simulink model "getAcceleration"  (R2019a)
settings: Solver=FixedStepAuto  StartTime=0.0  StopTime=inf  RelTol=1e-3  EnableMultiTasking=on
settings Model: SimulationMode=external  Creator=florian  LastModifiedBy=florian
settings SolverCC: PositivePriorityOrder=on
settings OptimizationCC: EnhancedBackFolding=on  PassReuseOutputArgsAs=Individual arguments  MaxStackSize=64  OptimizeBlockOrder=speed  DifferentSizesBufferReuse=on  OptimizationCustomize=off
settings DebuggingCC: ParameterTunabilityLossMsg=error
settings HardwareCC: ProdBitPerPointer=32  ProdBitPerSizeT=32  ProdBitPerPtrDiffT=32  ProdLargestAtomicInteger=Long  ProdLargestAtomicFloat=Double  ProdWordSize=32  ProdLongLongMode=on  ProdHWDeviceType=ARM Compatible->ARM Cortex
settings SFSimCC: MATLABDynamicMemAlloc=off
settings RTWCC: SystemTargetFile=ert.tlc  HardwareBoard=Raspberry Pi  TLCOptions="-aInlineSetEventsForThisBaseRateFcn=TLC_FALSE -aSuppressMultiTaskScheduler=TLC_FALSE  -aRateBasedStepFcn=0"  TemplateMakefile=ert_default_tmf  GenerateReport=on  Toolchain=GNU GCC Raspberry Pi  BuildConfiguration=Faster Runs  IncludeHyperlinkInReport=on  LaunchReport=on  GenerateTraceInfo=on  GenerateTraceReport=on  GenerateTraceReportSl=on  GenerateTraceReportSf=on  GenerateTraceReportEml=on
settings CodeAppCC: ForceParamTrailComments=on  IgnoreCustomStorageClasses=off  OperatorAnnotations=on  SimulinkDataObjDesc=on  SFDataObjDesc=on  InsertBlockDesc=on
settings ERTTargetCC: SupportContinuousTime=on  SupportVariableSizeSignals=on

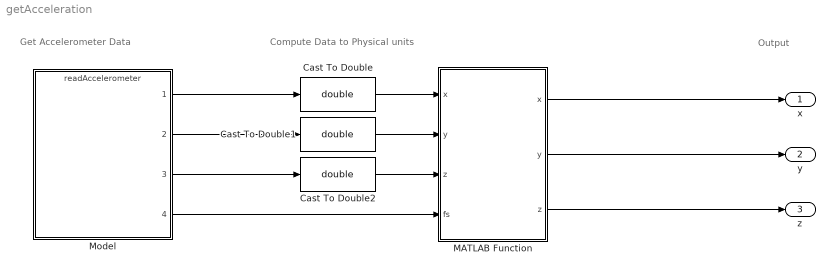
== system getAcceleration ==
  note: Compute Data to Physical units
  note: Output
  note: Get Accelerometer Data
  Cast To Double : DataTypeConversion  OutDataTypeStr=double
  Cast To Double1 : DataTypeConversion  OutDataTypeStr=double
  Cast To Double2 : DataTypeConversion  OutDataTypeStr=double
  MATLAB Function : MATLAB Function  TreatAsAtomicUnit=on
  Model : ModelReference  ModelNameDialog=readAccelerometer.slx  SimulationMode=Normal  ModelReferenceVersion=1.17
  x : Outport
  y : Outport  Port=2
  z : Outport  Port=3
  wires:
  Model/1 -> Cast To Double/1
  Model/2 -> Cast To Double1/1
  Model/3 -> Cast To Double2/1
  Model/4 -> MATLAB Function/4(fs)
  Cast To Double/1 -> MATLAB Function/1("x ")
  Cast To Double1/1 -> MATLAB Function/2("y ")
  Cast To Double2/1 -> MATLAB Function/3("z ")
  MATLAB Function/1(x) -> x/1
  MATLAB Function/2(y) -> y/1
  MATLAB Function/3(z) -> z/1

== matlab function getAcceleration/MATLAB Function ==
  data: x output; x input; y output; y input; z input; fs input; z output
function [x, y, z] = getPhysicalValues(x, y ,z, fs)
    % Compute Sensitivity in mg/LSB (Observation that this function equivalent to Table in Datasheet)
    sensitivity = fs/2*0.061;
    % Conventional value of earths acceleration in m/s^2
    g = 9.80665;
    % Compute the Data to m/s^2 (Sensitivity in mg/LSB -> *1000 -> g/LSB ->
    % *g -> m/s^2/LSB -> *value -> m/s^2
    x = x*sensitivity/1000*g;
    y = y*sensitivity/1000*g;
    z = z*sensitivity/1000*g;
